simulink model "Sensor_Temp"  (R2022b)
settings: Solver=VariableStepAuto  StartTime=0.0  StopTime=10.0  RelTol=1e-3
libraries: dspstat3 x1
settings Model: Creator=aceao  LastModifiedBy=aceao

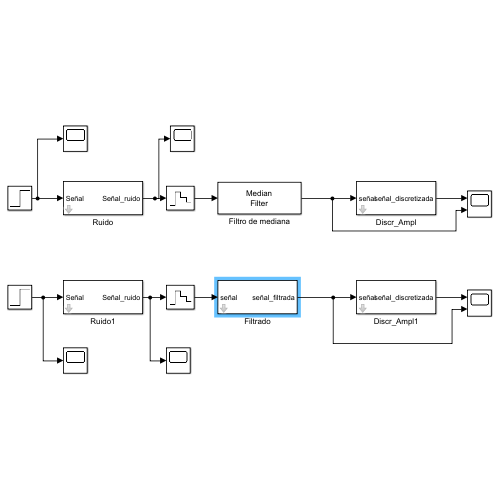
[thumbnail: Simulink's stored preview of the top-level diagram]
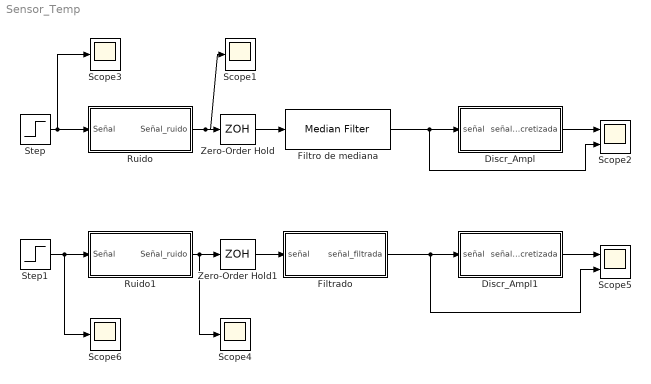
== system Sensor_Temp ==
  Discr_Ampl : Subsystem  mask{N=65536, Min=-40, Max=250}
      mask prompts: N "Valores distintos (N)"; Min "Valor mínimo"; Max "Valor máximo"
      mask DialogControl DescGroupVar Prompt: Discretizacion_Amplitud
      mask DialogControl DescTextVar Prompt: Discretización en amplitud
  Discr_Ampl1 : Subsystem  mask{N=65536, Min=-40, Max=250}
      mask prompts: N "Valores distintos (N)"; Min "Valor mínimo"; Max "Valor máximo"
      mask DialogControl DescGroupVar Prompt: Discretizacion_Amplitud
      mask DialogControl DescTextVar Prompt: Discretización en amplitud
  Filtrado : Subsystem  mask{error=1}
      mask prompts: error "Umbral error (ºC)"
      mask DialogControl DescGroupVar Prompt: Discretizacion_Amplitud
      mask DialogControl DescTextVar Prompt: Discretización en amplitud
  Filtro de mediana : dspstat3/Median Filter  WindowLength=4  SimulateUsing=Interpreted execution
      settings: LibrarySourceBlock=|
      | dspfdesign/Median
      | Filter
  Ruido : Subsystem  mask{M=0, V=0.3, T=0.15}
      mask prompts: M "Media"; V "Varianza"; T "Periodo"
      mask DialogControl Ruido Prompt: Ruido
      mask DialogControl DescTextVar Prompt: Añade ruido gaussiano
  Ruido1 : Subsystem  mask{M=0, V=0.3, T=0.15}
      mask prompts: M "Media"; V "Varianza"; T "Periodo"
      mask DialogControl Ruido Prompt: Ruido
      mask DialogControl DescTextVar Prompt: Añade ruido gaussiano
  Scope{1,3..4,6} (4 alike) : Scope
  Scope2 : Scope  NumInputPorts=2
  Scope5 : Scope  NumInputPorts=2
  Step : Step  Before=40  After=45  SampleTime=0
  Step1 : Step  Before=40  After=45  SampleTime=0
  Zero-Order Hold : ZeroOrderHold  SampleTime=0.15
  Zero-Order Hold1 : ZeroOrderHold  SampleTime=0.15
  wires:
  Step/1 -> Scope3/1, Ruido/1(Señal)
  Ruido/1(Señal_ruido) -> Scope1/1, Zero-Order Hold/1
  Zero-Order Hold/1 -> Filtro de mediana/1
  Filtro de mediana/1 -> Discr_Ampl/1(señal), Scope2/2
  Discr_Ampl/1(señal_discretizada) -> Scope2/1
  Filtrado/1(señal_filtrada) -> Scope5/2, Discr_Ampl1/1(señal)
  Ruido1/1(Señal_ruido) -> Scope4/1, Zero-Order Hold1/1
  Zero-Order Hold1/1 -> Filtrado/1(señal)
  Discr_Ampl1/1(señal_discretizada) -> Scope5/1
  Step1/1 -> Scope6/1, Ruido1/1(Señal)

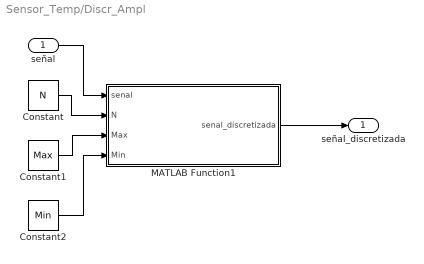
== system Sensor_Temp/Discr_Ampl ==
  señal : Inport
  Constant : Constant  Value=N
  Constant1 : Constant  Value=Max
  Constant2 : Constant  Value=Min
  MATLAB Function1 : MATLAB Function  TreatAsAtomicUnit=on
  señal_discretizada : Outport
  wires:
  MATLAB Function1/1(senal_discretizada) -> señal_discretizada/1
  señal/1 -> MATLAB Function1/1(senal)
  Constant1/1 -> MATLAB Function1/3(Max)
  Constant/1 -> MATLAB Function1/2(N)
  Constant2/1 -> MATLAB Function1/4(Min)

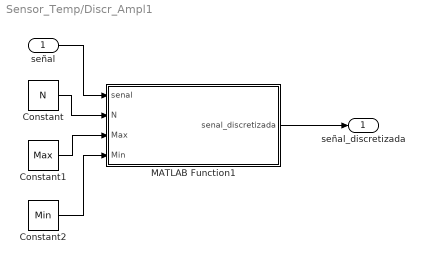
== system Sensor_Temp/Discr_Ampl1 ==
  señal : Inport
  Constant : Constant  Value=N
  Constant1 : Constant  Value=Max
  Constant2 : Constant  Value=Min
  MATLAB Function1 : MATLAB Function  TreatAsAtomicUnit=on
  señal_discretizada : Outport
  wires:
  MATLAB Function1/1(senal_discretizada) -> señal_discretizada/1
  señal/1 -> MATLAB Function1/1(senal)
  Constant1/1 -> MATLAB Function1/3(Max)
  Constant/1 -> MATLAB Function1/2(N)
  Constant2/1 -> MATLAB Function1/4(Min)

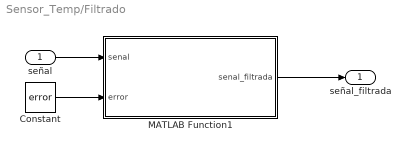
== system Sensor_Temp/Filtrado ==
  señal : Inport
  Constant : Constant  Value=error
  MATLAB Function1 : MATLAB Function  TreatAsAtomicUnit=on
  señal_filtrada : Outport
  wires:
  MATLAB Function1/1(senal_filtrada) -> señal_filtrada/1
  señal/1 -> MATLAB Function1/1(senal)
  Constant/1 -> MATLAB Function1/2(error)

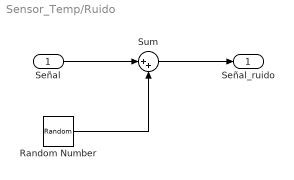
== system Sensor_Temp/Ruido ==
  Señal : Inport
  Random Number : RandomNumber  Mean=M  Variance=V  Seed=2  SampleTime=T
  Sum : Sum  Inputs=|++
  Señal_ruido : Outport
  wires:
  Random Number/1 -> Sum/2
  Señal/1 -> Sum/1
  Sum/1 -> Señal_ruido/1

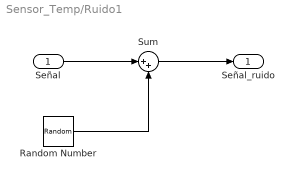
== system Sensor_Temp/Ruido1 ==
  Señal : Inport
  Random Number : RandomNumber  Mean=M  Variance=V  Seed=2  SampleTime=T
  Sum : Sum  Inputs=|++
  Señal_ruido : Outport
  wires:
  Random Number/1 -> Sum/2
  Señal/1 -> Sum/1
  Sum/1 -> Señal_ruido/1

== matlab function Sensor_Temp/Discr_Ampl/MATLAB Function1 ==
  data: senal input; senal_discretizada output; N input; Max input; Min input
function senal_discretizada  = fcn(senal,N,Max,Min)

if(senal>Max)
    senal_discretizada=Max;
    return
elseif(senal<Min)
    senal_discretizada=Min;
    return
end

valor_escalon=(Max-Min)/(N-1);
i=Min;
 while(i<Max)
    if(i+valor_escalon/2>senal)
        senal_discretizada=i;
        return
    end
    i=i+valor_escalon;
end

      senal_discretizada=Max;
end

== matlab function Sensor_Temp/Discr_Ampl1/MATLAB Function1 ==
  data: senal input; senal_discretizada output; N input; Max input; Min input
function senal_discretizada  = fcn(senal,N,Max,Min)

if(senal>Max)
    senal_discretizada=Max;
    return
elseif(senal<Min)
    senal_discretizada=Min;
    return
end

valor_escalon=(Max-Min)/(N-1);
i=Min;
 while(i<Max)
    if(i+valor_escalon/2>senal)
        senal_discretizada=i;
        return
    end
    i=i+valor_escalon;
end

      senal_discretizada=Max;
end

== matlab function Sensor_Temp/Filtrado/MATLAB Function1 ==
  data: senal input; senal_filtrada output; error input
function senal_filtrada  = fcn(senal,error)


end
